simulink model "kuka_classic_mda_daan_carthesian"  (R2014b)
settings: Solver=ode4  StartTime=0  StopTime=r.t(end)  FixedStep=r.t(2) - r.t(1)  RelTol=1e-3
undefined symbols (not defined in the file or in its folder): cyl0, r_n, z
libraries: simulink x1
settings Model: Creator=dpool  LastModifiedBy=fdrop
settings DataIOCC: SignalLoggingSaveFormat=ModelDataLogs
settings OptimizationCC: ExpressionDepthLimit=2147483647
settings DebuggingCC: UnderspecifiedInitializationDetection=Classic  MergeDetectMultiDrivingBlocksExec=none  FcnCallInpInsideContextMsg=EnableAllAsWarning  StateNameClashWarn=warning

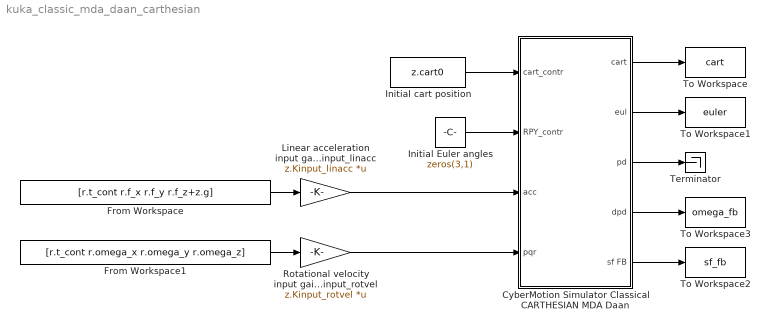
== system kuka_classic_mda_daan_carthesian ==
  CyberMotion Simulator Classical CARTHESIAN MDA Daan : Subsystem
  From Workspace : FromWorkspace  VariableName=[r.t_cont r.f_x r.f_y r.f_z+z.g]  SampleTime=0
  From Workspace1 : FromWorkspace  VariableName=[r.t_cont r.omega_x r.omega_y r.omega_z]  SampleTime=0
  Initial Euler angles : Constant  Value=zeros(3,1)
  Initial cart position : Constant  Value=z.cart0
  Linear acceleration input gain: Kinput_linacc : Gain  Gain=z.Kinput_linacc  Multiplication=Matrix(K*u)
  Rotational velocity input gain: Kinput_rotvel : Gain  Gain=z.Kinput_rotvel  Multiplication=Matrix(K*u)
  Terminator : Terminator
  To Workspace : ToWorkspace  VariableName=cart  SampleTime=-1
      settings: Save2DSignal=2-D array (concatenate along first dimension)
  To Workspace1 : ToWorkspace  VariableName=euler  SampleTime=-1
  To Workspace2 : ToWorkspace  VariableName=sf_fb  SampleTime=-1
  To Workspace3 : ToWorkspace  VariableName=omega_fb  SampleTime=-1
  wires:
  From Workspace/1 -> Linear acceleration input gain: Kinput_linacc/1
  From Workspace1/1 -> Rotational velocity input gain: Kinput_rotvel/1
  Initial cart position/1 -> CyberMotion Simulator Classical CARTHESIAN MDA Daan/1(cart_contr)
  Linear acceleration input gain: Kinput_linacc/1 -> CyberMotion Simulator Classical CARTHESIAN MDA Daan/3(acc)
  Rotational velocity input gain: Kinput_rotvel/1 -> CyberMotion Simulator Classical CARTHESIAN MDA Daan/4(pqr)
  Initial Euler angles/1 -> CyberMotion Simulator Classical CARTHESIAN MDA Daan/2(RPY_contr)
  CyberMotion Simulator Classical CARTHESIAN MDA Daan/1(cart) -> To Workspace/1
  CyberMotion Simulator Classical CARTHESIAN MDA Daan/2(eul) -> To Workspace1/1
  CyberMotion Simulator Classical CARTHESIAN MDA Daan/3(pd) -> Terminator/1
  CyberMotion Simulator Classical CARTHESIAN MDA Daan/4(dpd) -> To Workspace3/1
  CyberMotion Simulator Classical CARTHESIAN MDA Daan/5(sf FB) -> To Workspace2/1

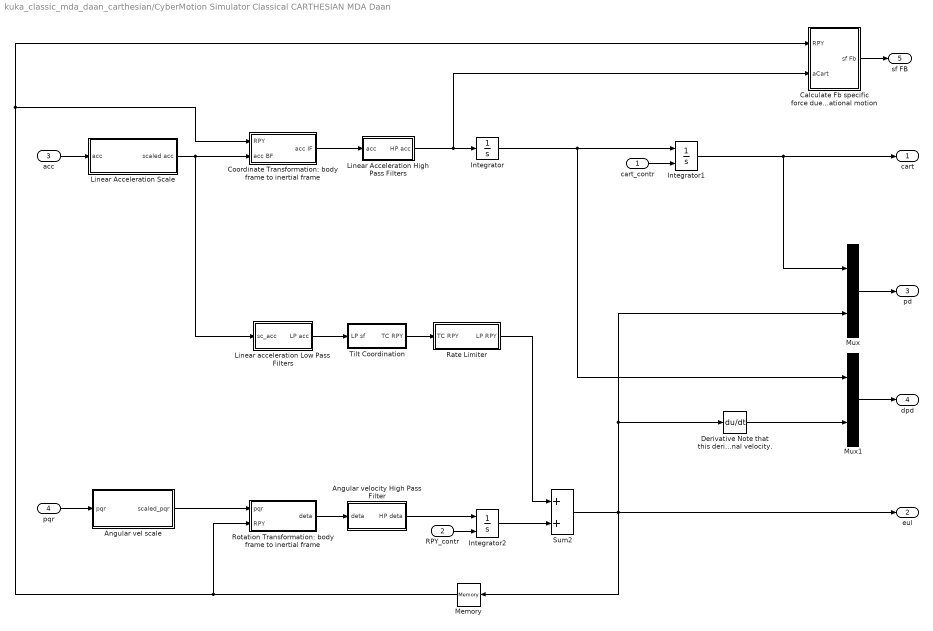
== system kuka_classic_mda_daan_carthesian/CyberMotion Simulator Classical CARTHESIAN MDA Daan ==
  cart_contr : Inport
  RPY_contr : Inport  Port=2
  acc : Inport  Port=3
  pqr : Inport  Port=4
  " Linear Acceleration High Pass Filters" : Subsystem
  Angular vel scale : Subsystem
  Angular velocity High Pass Filter : Subsystem
  Calculate Fb specific force due to commanded MDA linear and rotational motion : Subsystem
  Coordinate Transformation: body frame to inertial frame : Subsystem
  Derivative Note that this derivative block is needed to incorporate the effect of the tilt coordination channel on the rotational velocity. : Derivative
  Integrator : Integrator
  Integrator1 : Integrator  InitialConditionSource=external  InitialCondition=cyl0
  Integrator2 : Integrator  InitialConditionSource=external
  Linear Acceleration Scale : Subsystem
  Linear acceleration Low Pass Filters : Subsystem
  Memory : Memory
  Mux : Mux  Inputs=2
  Mux1 : Mux  Inputs=2
  Rate Limiter : Subsystem
  Rotation Transformation: body frame to inertial frame : Subsystem
  Sum2 : Sum  SaturateOnIntegerOverflow=on
  Tilt Coordination : Subsystem
  cart : Outport
  eul : Outport  Port=2
  pd : Outport  Port=3
  dpd : Outport  Port=4
  sf FB : Outport  Port=5
  wires:
  Mux/1 -> pd/1
  Mux1/1 -> dpd/1
  Derivative Note that this derivative block is needed to incorporate the effect of the tilt coordination channel on the rotational velocity./1 -> Mux1/2
  Angular velocity High Pass Filter/1(HP deta) -> Integrator2/1
  pqr/1 -> Angular vel scale/1(pqr)
  " Linear Acceleration High Pass Filters"/1(HP acc) -> Integrator/1, Calculate Fb specific force due to commanded MDA linear and rotational motion/2(aCart)
  Linear Acceleration Scale/1(scaled acc) -> Linear acceleration Low Pass Filters/1(sc_acc), Coordinate Transformation: body frame to inertial frame/2(acc BF)
  Integrator/1 -> Integrator1/1, Mux1/1
  Integrator1/1 -> cart/1, Mux/1
  Tilt Coordination/1(TC RPY) -> Rate Limiter/1(TC RPY)
  acc/1 -> Linear Acceleration Scale/1(acc)
  Sum2/1 -> eul/1, Memory/1, Derivative Note that this derivative block is needed to incorporate the effect of the tilt coordination channel on the rotational velocity./1, Mux/2
  Memory/1 -> Rotation Transformation: body frame to inertial frame/2(RPY), Coordinate Transformation: body frame to inertial frame/1(RPY), Calculate Fb specific force due to commanded MDA linear and rotational motion/1(RPY)
  Integrator2/1 -> Sum2/2
  Rate Limiter/1(LP RPY) -> Sum2/1
  Angular vel scale/1(scaled_pqr) -> Rotation Transformation: body frame to inertial frame/1(pqr)
  Rotation Transformation: body frame to inertial frame/1(deta) -> Angular velocity High Pass Filter/1(deta)
  cart_contr/1 -> Integrator1/2
  RPY_contr/1 -> Integrator2/2
  Linear acceleration Low Pass Filters/1(LP acc) -> Tilt Coordination/1(LP sf)
  Calculate Fb specific force due to commanded MDA linear and rotational motion/1(sf Fb) -> sf FB/1
  Coordinate Transformation: body frame to inertial frame/1(acc IF) -> " Linear Acceleration High Pass Filters"/1(acc)

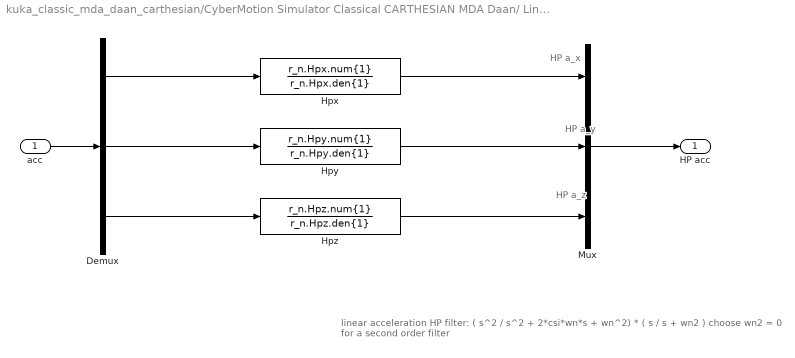
== system kuka_classic_mda_daan_carthesian/CyberMotion Simulator Classical CARTHESIAN MDA Daan/ Linear Acceleration High Pass Filters ==
  note: HP a_x
  note: HP a_y
  note: HP a_z
  note: linear acceleration HP filter:  ( s^2 / s^2 + 2*csi*wn*s + wn^2) * ( s / s + wn2 )
      | choose wn2 = 0 for a second order filter
  acc : Inport
  Demux : Demux  Outputs=3
  Hpx : TransferFcn  Numerator=r_n.Hpx.num{1}  Denominator=r_n.Hpx.den{1}
  Hpy : TransferFcn  Numerator=r_n.Hpy.num{1}  Denominator=r_n.Hpy.den{1}
  Hpz : TransferFcn  Numerator=r_n.Hpz.num{1}  Denominator=r_n.Hpz.den{1}
  Mux : Mux  Inputs=3
  HP acc : Outport
  wires:
  Demux/1 -> Hpx/1
  Demux/2 -> Hpy/1
  Demux/3 -> Hpz/1
  acc/1 -> Demux/1
  Hpx/1 -> Mux/1
  Hpy/1 -> Mux/2
  Mux/1 -> HP acc/1
  Hpz/1 -> Mux/3

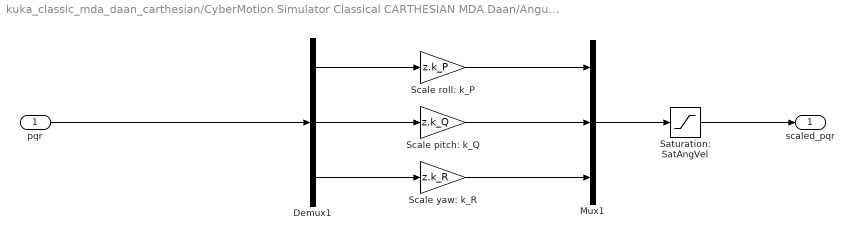
== system kuka_classic_mda_daan_carthesian/CyberMotion Simulator Classical CARTHESIAN MDA Daan/Angular vel scale ==
  pqr : Inport
  Demux1 : Demux  Outputs=3
  Mux1 : Mux  Inputs=3
  Saturation: SatAngVel : Saturate  UpperLimit=z.SatAngVel  LowerLimit=-z.SatAngVel
  Scale pitch: k_Q : Gain  Gain=z.k_Q  SaturateOnIntegerOverflow=on  OutDataTypeStr=Inherit: Same as input  ParamDataTypeStr=Inherit: Same as input
  Scale roll: k_P : Gain  Gain=z.k_P  SaturateOnIntegerOverflow=on  OutDataTypeStr=Inherit: Same as input  ParamDataTypeStr=Inherit: Same as input
  Scale yaw: k_R : Gain  Gain=z.k_R  SaturateOnIntegerOverflow=on  OutDataTypeStr=Inherit: Same as input  ParamDataTypeStr=Inherit: Same as input
  scaled_pqr : Outport
  wires:
  Scale roll: k_P/1 -> Mux1/1
  Scale pitch: k_Q/1 -> Mux1/2
  Mux1/1 -> Saturation: SatAngVel/1
  Scale yaw: k_R/1 -> Mux1/3
  Demux1/1 -> Scale roll: k_P/1
  Demux1/2 -> Scale pitch: k_Q/1
  Demux1/3 -> Scale yaw: k_R/1
  pqr/1 -> Demux1/1
  Saturation: SatAngVel/1 -> scaled_pqr/1

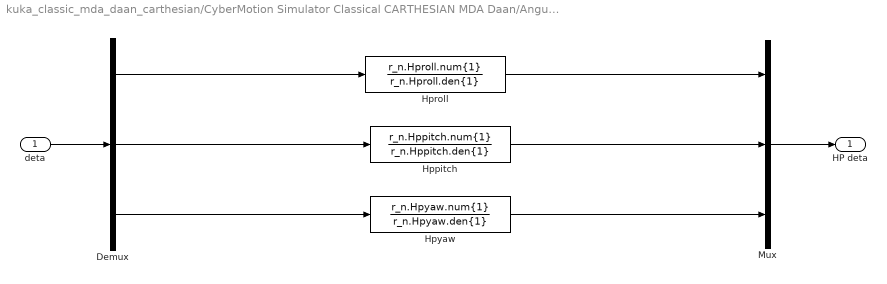
== system kuka_classic_mda_daan_carthesian/CyberMotion Simulator Classical CARTHESIAN MDA Daan/Angular velocity High Pass Filter ==
  deta : Inport
  Demux : Demux  Outputs=3
  Hppitch : TransferFcn  Numerator=r_n.Hppitch.num{1}  Denominator=r_n.Hppitch.den{1}
  Hproll : TransferFcn  Numerator=r_n.Hproll.num{1}  Denominator=r_n.Hproll.den{1}
  Hpyaw : TransferFcn  Numerator=r_n.Hpyaw.num{1}  Denominator=r_n.Hpyaw.den{1}
  Mux : Mux  Inputs=3
  HP deta : Outport
  wires:
  Hppitch/1 -> Mux/2
  Hproll/1 -> Mux/1
  Demux/1 -> Hproll/1
  Demux/2 -> Hppitch/1
  deta/1 -> Demux/1
  Demux/3 -> Hpyaw/1
  Hpyaw/1 -> Mux/3
  Mux/1 -> HP deta/1

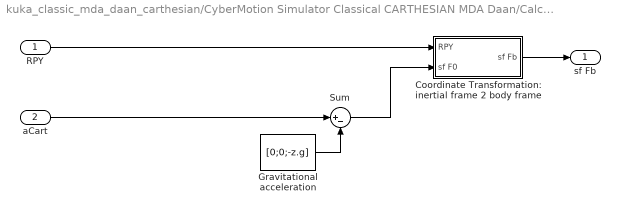
== system kuka_classic_mda_daan_carthesian/CyberMotion Simulator Classical CARTHESIAN MDA Daan/Calculate Fb specific force due to commanded MDA linear and rotational motion ==
  RPY : Inport
  aCart : Inport  Port=2
  Coordinate Transformation: inertial frame 2 body frame : Subsystem
  Gravitational acceleration : Constant  Value=[0;0;-z.g]
  Sum : Sum  Inputs=|+-
  sf Fb : Outport
  wires:
  RPY/1 -> Coordinate Transformation: inertial frame 2 body frame/1(RPY)
  Coordinate Transformation: inertial frame 2 body frame/1(sf Fb) -> sf Fb/1
  Sum/1 -> Coordinate Transformation: inertial frame 2 body frame/2(sf F0)
  Gravitational acceleration/1 -> Sum/2
  aCart/1 -> Sum/1

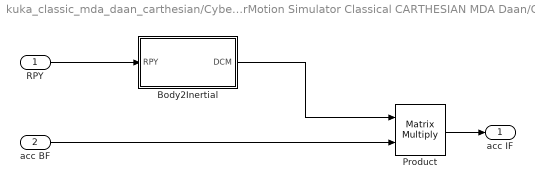
== system kuka_classic_mda_daan_carthesian/CyberMotion Simulator Classical CARTHESIAN MDA Daan/Coordinate Transformation: body frame to inertial frame ==
  RPY : Inport
  acc BF : Inport  Port=2
  Body2Inertial : MATLAB Function  TreatAsAtomicUnit=on
  Product : Product  Multiplication=Matrix(*)  RndMeth=Zero
  acc IF : Outport
  wires:
  acc BF/1 -> Product/2
  Product/1 -> acc IF/1
  RPY/1 -> Body2Inertial/1(RPY)
  Body2Inertial/1(DCM) -> Product/1

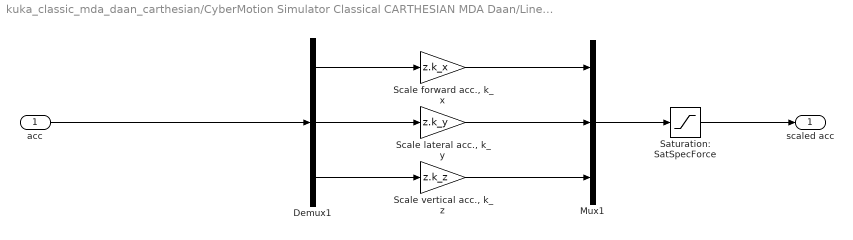
== system kuka_classic_mda_daan_carthesian/CyberMotion Simulator Classical CARTHESIAN MDA Daan/Linear Acceleration Scale ==
  acc : Inport
  Demux1 : Demux  Outputs=3
  Mux1 : Mux  Inputs=3
  Saturation: SatSpecForce : Saturate  UpperLimit=z.SatSpecForce  LowerLimit=-z.SatSpecForce
  "Scale forward acc., k_x" : Gain  Gain=z.k_x  SaturateOnIntegerOverflow=on  OutDataTypeStr=Inherit: Same as input  ParamDataTypeStr=Inherit: Same as input
  "Scale lateral acc., k_y" : Gain  Gain=z.k_y  SaturateOnIntegerOverflow=on  OutDataTypeStr=Inherit: Same as input  ParamDataTypeStr=Inherit: Same as input
  "Scale vertical acc., k_z" : Gain  Gain=z.k_z  SaturateOnIntegerOverflow=on  OutDataTypeStr=Inherit: Same as input  ParamDataTypeStr=Inherit: Same as input
  scaled acc : Outport
  wires:
  "Scale forward acc., k_x"/1 -> Mux1/1
  "Scale lateral acc., k_y"/1 -> Mux1/2
  Mux1/1 -> Saturation: SatSpecForce/1
  "Scale vertical acc., k_z"/1 -> Mux1/3
  Demux1/1 -> "Scale forward acc., k_x"/1
  Demux1/2 -> "Scale lateral acc., k_y"/1
  Demux1/3 -> "Scale vertical acc., k_z"/1
  acc/1 -> Demux1/1
  Saturation: SatSpecForce/1 -> scaled acc/1

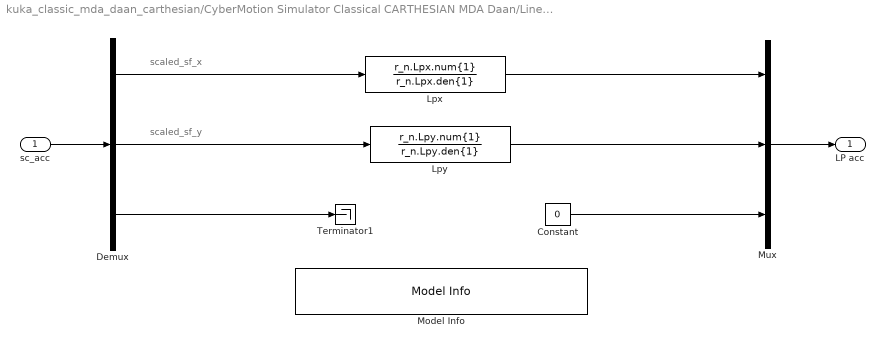
== system kuka_classic_mda_daan_carthesian/CyberMotion Simulator Classical CARTHESIAN MDA Daan/Linear acceleration Low Pass Filters ==
  note: scaled_sf_x
  note: scaled_sf_y
  sc_acc : Inport
  Constant : Constant  Value=0
  Demux : Demux  Outputs=3
  Lpx : TransferFcn  Numerator=r_n.Lpx.num{1}  Denominator=r_n.Lpx.den{1}
  Lpy : TransferFcn  Numerator=r_n.Lpy.num{1}  Denominator=r_n.Lpy.den{1}
  Model Info : simulink/Model-Wide Utilities/Model Info  BlockCM=None  Frame=on  DisplayStringWithTags=|  HorizontalTextAlignment=Center  LeftAlignmentValue=0.5  SourceBlockDiagram=kuka_classic_mda_daan_carthesian  TagMaxNumber=20
      | Tilt coordination can only be performed for pitch
      | and roll. Hence, the yaw channel here always
      | outputs zero.
  Mux : Mux  Inputs=3
  Terminator1 : Terminator
  LP acc : Outport
  wires:
  Lpy/1 -> Mux/2
  Lpx/1 -> Mux/1
  Demux/1 -> Lpx/1
  Demux/2 -> Lpy/1
  sc_acc/1 -> Demux/1
  Demux/3 -> Terminator1/1
  Constant/1 -> Mux/3
  Mux/1 -> LP acc/1

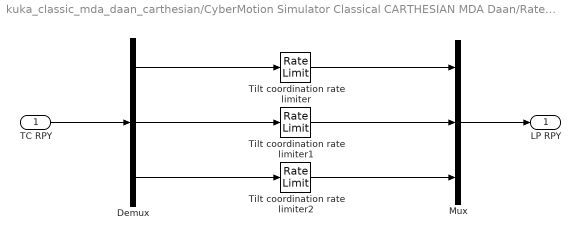
== system kuka_classic_mda_daan_carthesian/CyberMotion Simulator Classical CARTHESIAN MDA Daan/Rate Limiter ==
  TC RPY : Inport
  Demux : Demux  Outputs=3
  Mux : Mux  Inputs=3
  Tilt coordination rate limiter : RateLimiter  RisingSlewLimit=z.TC_ratelimit  FallingSlewLimit=-z.TC_ratelimit  SampleTimeMode=inherited
  Tilt coordination rate limiter1 : RateLimiter  RisingSlewLimit=z.TC_ratelimit  FallingSlewLimit=-z.TC_ratelimit  SampleTimeMode=inherited
  Tilt coordination rate limiter2 : RateLimiter  RisingSlewLimit=z.TC_ratelimit  FallingSlewLimit=-z.TC_ratelimit  SampleTimeMode=inherited
  LP RPY : Outport
  wires:
  TC RPY/1 -> Demux/1
  Demux/1 -> Tilt coordination rate limiter/1
  Demux/2 -> Tilt coordination rate limiter1/1
  Demux/3 -> Tilt coordination rate limiter2/1
  Mux/1 -> LP RPY/1
  Tilt coordination rate limiter/1 -> Mux/1
  Tilt coordination rate limiter1/1 -> Mux/2
  Tilt coordination rate limiter2/1 -> Mux/3

== system kuka_classic_mda_daan_carthesian/CyberMotion Simulator Classical CARTHESIAN MDA Daan/Rotation Transformation: body frame to inertial frame ==
  pqr : Inport
  RPY : Inport  Port=2
  "Body2Inertial: Rotations Eq. (2.12), Reid 1985" : MATLAB Function  TreatAsAtomicUnit=on
  Product : Product  Multiplication=Matrix(*)  RndMeth=Zero
  deta : Outport
  wires:
  pqr/1 -> Product/2
  Product/1 -> deta/1
  RPY/1 -> "Body2Inertial: Rotations Eq. (2.12), Reid 1985"/1(RPY)
  "Body2Inertial: Rotations Eq. (2.12), Reid 1985"/1(DCM) -> Product/1

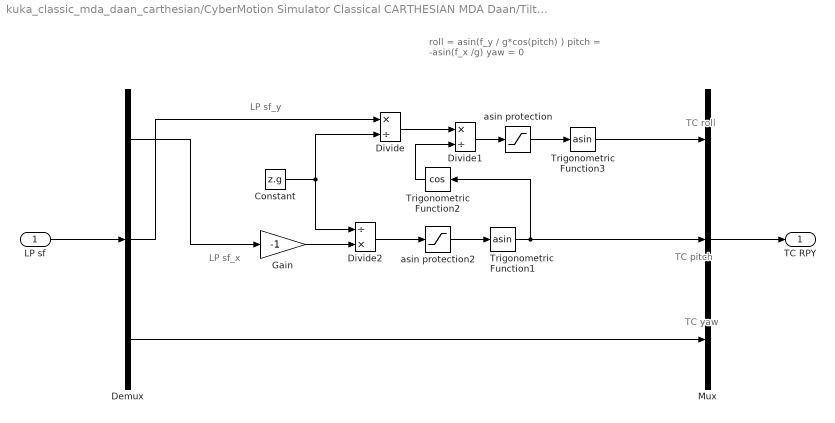
== system kuka_classic_mda_daan_carthesian/CyberMotion Simulator Classical CARTHESIAN MDA Daan/Tilt Coordination ==
  note: TC roll
  note: TC pitch
  note: TC yaw
  note: roll     =    asin(f_y / g*cos(pitch)  )
      | pitch  =    -asin(f_x /g)
      | yaw   =     0
  note: LP sf_y
  note: LP sf_x
  LP sf : Inport
  Constant : Constant  Value=z.g
  Demux : Demux  Outputs=3
  Divide : Product  Inputs=*/
  Divide1 : Product  Inputs=*/
  Divide2 : Product  Inputs=/*
  Gain : Gain  Gain=-1
  Mux : Mux  Inputs=3
  Trigonometric Function1 : Trigonometry  Operator=asin
  Trigonometric Function2 : Trigonometry  Operator=cos
  Trigonometric Function3 : Trigonometry  Operator=asin
  asin protection : Saturate  UpperLimit=1  LowerLimit=-1
  asin protection2 : Saturate  UpperLimit=1  LowerLimit=-1
  TC RPY : Outport
  wires:
  Demux/3 -> Mux/3
  Mux/1 -> TC RPY/1
  Divide/1 -> Divide1/1
  Divide1/1 -> asin protection/1
  asin protection/1 -> Trigonometric Function3/1
  Trigonometric Function3/1 -> Mux/1
  Constant/1 -> Divide2/1, Divide/2
  Divide2/1 -> asin protection2/1
  asin protection2/1 -> Trigonometric Function1/1
  Trigonometric Function1/1 -> Trigonometric Function2/1, Mux/2
  Trigonometric Function2/1 -> Divide1/2
  Gain/1 -> Divide2/2
  Demux/1 -> Gain/1
  Demux/2 -> Divide/1
  LP sf/1 -> Demux/1

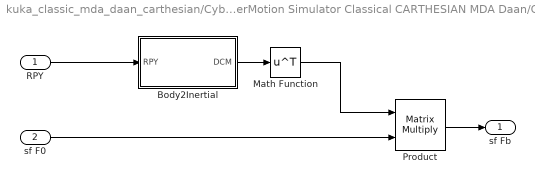
== system kuka_classic_mda_daan_carthesian/CyberMotion Simulator Classical CARTHESIAN MDA Daan/Calculate Fb specific force due to commanded MDA linear and rotational motion/Coordinate Transformation: inertial frame 2 body frame ==
  RPY : Inport
  sf F0 : Inport  Port=2
  Body2Inertial : MATLAB Function  TreatAsAtomicUnit=on
  Math Function : Math  Operator=transpose  SaturateOnIntegerOverflow=on
  Product : Product  Multiplication=Matrix(*)  RndMeth=Zero
  sf Fb : Outport
  wires:
  Math Function/1 -> Product/1
  Body2Inertial/1(DCM) -> Math Function/1
  RPY/1 -> Body2Inertial/1(RPY)
  Product/1 -> sf Fb/1
  sf F0/1 -> Product/2

== matlab function kuka_classic_mda_daan_carthesian/CyberMotion Simulator Classical CARTHESIAN MDA Daan/Coordinate Transformation: body frame to inertial frame/Body2Inertial ==
  data: RPY input; DCM output
function DCM = BF2IF(RPY)
% This block supports the Embedded MATLAB subset.
% See the help menu for details. 

r = RPY(1);
p = RPY(2);
y = RPY(3);
RPYrot = [ cos(y)*cos(p)  cos(y)*sin(p)*sin(r)-sin(y)*cos(r)  cos(y)*sin(p)*cos(r)+sin(y)*sin(r);
          sin(y)*cos(p)  sin(y)*sin(p)*sin(r)+cos(y)*cos(r)  sin(y)*sin(p)*cos(r)-cos(y)*sin(r);
             -sin(p)                  cos(p)*sin(r)                      cos(p)*cos(r)];

DCM = RPYrot;

== matlab function kuka_classic_mda_daan_carthesian/CyberMotion Simulator Classical CARTHESIAN MDA Daan/Rotation Transformation: body frame to inertial frame/Body2Inertial: Rotations Eq. (2.12), Reid 1985 ==
  data: RPY input; DCM output
function DCM = BF2IF_ROT(RPY)

% Rotation matrix that can be used to convert rotational velocities
% expressed in body axes (pqr) to corresponding inertial Euler rates. This
% rotation matrix is defined as Eq. (2.12) in [Reid & Nahon, 1985], p. 2.4.
%
% Daan Pool
% October 2012

% retrieve roll and pitch attitude
r = RPY(1);
p = RPY(2);
% y = RPY(3);
         
% construct rotation matrix
DCM = [ 1  sin(r)*tan(p)  cos(r)*tan(p) ;
        0  cos(r)        -sin(r)        ;
        0  sin(r)/cos(p)  cos(r)/cos(p) ];

== matlab function kuka_classic_mda_daan_carthesian/CyberMotion Simulator Classical CARTHESIAN MDA Daan/Calculate Fb specific force due to commanded MDA linear and rotational motion/Coordinate Transformation: inertial frame 2 body frame/Body2Inertial ==
  data: RPY input; DCM output
function DCM = BF2IF(RPY)
% This block supports the Embedded MATLAB subset.
% See the help menu for details. 

r = RPY(1);
p = RPY(2);
y = RPY(3);
RPYrot = [ cos(y)*cos(p)  cos(y)*sin(p)*sin(r)-sin(y)*cos(r)  cos(y)*sin(p)*cos(r)+sin(y)*sin(r);
          sin(y)*cos(p)  sin(y)*sin(p)*sin(r)+cos(y)*cos(r)  sin(y)*sin(p)*cos(r)-cos(y)*sin(r);
             -sin(p)                  cos(p)*sin(r)                      cos(p)*cos(r)];

DCM = RPYrot;
